simulink model "chou1"  (Simulink 2.09)
settings: Solver=ode45  StartTime=0.0  StopTime=9999  MaxStep=0.001  RelTol=1e-5  AbsTol=1e-5
settings Model: SaveTime=off  SaveOutput=off  ConsistencyChecking=off  RTWTemplateMakefile=grt_vc.tmf

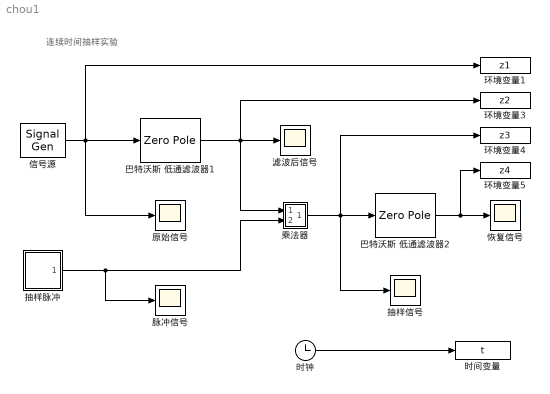
== system chou1 ==
  note: 连续时间抽样实验
  巴特沃斯 低通滤波器1 : ZeroPole  Zeros=z  Poles=p  Gain=k  mask(buttap){@1=60, @2=4}
      mask prompts: @1 "Cutoff frequency (rad/sec)"; @2 "Order"
      mask help:
      | Analog Butterworth low pass filter.
      |
      | (Requires Signal Processing Toolbox)
      mask init:
      | [z,p,k]=buttap(@2); z=@1*z; p=@1*p; k=real(prod(-p)); [num,den]=zp2tf(z,p,k); w=logspace(log10(@1/10),log10(10*@1),20); h=freqs(num,den,w);
      mask Help: Butterworth low pass filter using MATLAB's butter command.
      mask Display: plot(20*log10(w),20*log10(abs(h)))
  巴特沃斯 低通滤波器2 : ZeroPole  Zeros=z  Poles=p  Gain=k  mask(buttap){@1=60, @2=4}
      mask prompts: @1 "Cutoff frequency (rad/sec)"; @2 "Order"
      mask help:
      | Analog Butterworth low pass filter.
      |
      | (Requires Signal Processing Toolbox)
      mask init:
      | [z,p,k]=buttap(@2); z=@1*z; p=@1*p; k=real(prod(-p)); [num,den]=zp2tf(z,p,k); w=logspace(log10(@1/10),log10(10*@1),20); h=freqs(num,den,w);
      mask Help: Butterworth low pass filter using MATLAB's butter command.
      mask Display: plot(20*log10(w),20*log10(abs(h)))
  乘法器 : Subsystem
      mask Type: Dot Product
      mask Description:
      | Inner (dot) product.
      | y=sum(u1.*u2)
      mask Help: Computes the inner (dot) product of the inputs: sum(u1.*u2).  The inputs are vectors of the same length. Output is a scalar.
      mask Display: disp('X')
  抽样脉冲 : Subsystem  mask(Pulse Generator){@1=pi/100, @2=0.001, @3=1, @4=0.5}
      mask prompts: @1 "Pulse period (secs):"; @2 "Pulse width:"; @3 "Pulse height:"; @4 "Pulse start time:"
      mask help: Pulse Generator.
      mask init:
      | Ts=@1; du=@2; ht=@3; stt=@4; ini=ones(length(ht),1); st1=rem(stt,Ts); st2=rem(stt+du,Ts);if(Ts<=1.2*du),ini=zeros(length(ht),1);end;
      mask Help: Pulse generator which ensures pulse\ntransitions are hit. Provides a vector of pulses when the height is entered as a vector.\nUnmask to see how it works.
      mask Display: plot(0,0,100,100,[90,75,75,60,60,35,35,20,20,10],[20,20,80,80,20,20,80,80,20,20])
  抽样信号 : Scope
      settings: TickLabels=on  TimeRange=5  YMin=-2.6048  YMax=2.6048  SaveToWorkspace=off  SaveName=ScopeData
  环境变量1 : ToWorkspace  VariableName=z1  SampleTime=0
      settings: Buffer=1024*2
  环境变量3 : ToWorkspace  VariableName=z2  SampleTime=0
      settings: Buffer=1024*2
  环境变量4 : ToWorkspace  VariableName=z3  SampleTime=0
      settings: Buffer=1024*2
  环境变量5 : ToWorkspace  VariableName=z4  SampleTime=0
      settings: Buffer=1024*2
  恢复信号 : Scope
      settings: TickLabels=on  TimeRange=5  YMin=-0.108928  YMax=0.108928  SaveToWorkspace=off  SaveName=ScopeData
  滤波后信号 : Scope
      settings: TickLabels=on  TimeRange=5  YMin=-2.58112  YMax=2.58112  SaveToWorkspace=off  SaveName=ScopeData
  脉冲信号 : Scope
      settings: TickLabels=on  TimeRange=1  YMin=-1.55104  YMax=1.55104  SaveToWorkspace=off  SaveName=ScopeData
  时间变量 : ToWorkspace  VariableName=t  SampleTime=0
      settings: Buffer=2048
  时钟 : Clock
  信号源 : SignalGenerator  WaveForm=sine  Amplitude=2.000000  Frequency=3.140000  Units=rad/sec
  原始信号 : Scope
      settings: TickLabels=on  TimeRange=5  YMin=-4  YMax=4  SaveToWorkspace=off  SaveName=ScopeData
  wires:
  时钟/1 -> 时间变量/1
  巴特沃斯 低通滤波器2/1 -> 环境变量5/1, 恢复信号/1
  抽样脉冲/1(out_1) -> 脉冲信号/1, 乘法器/2(in_2)
  乘法器/1(out_1) -> 环境变量4/1, 抽样信号/1, 巴特沃斯 低通滤波器2/1
  巴特沃斯 低通滤波器1/1 -> 环境变量3/1, 滤波后信号/1, 乘法器/1(in_1)
  信号源/1 -> 环境变量1/1, 原始信号/1, 巴特沃斯 低通滤波器1/1

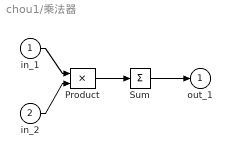
== system chou1/乘法器 ==
  in_1 : Inport  Port=1  PortWidth=-1  SampleTime=-1
  in_2 : Inport  Port=2  PortWidth=-1  SampleTime=-1
  Product : Product  Inputs=2
  Sum : Sum  Inputs=+
  out_1 : Outport  Port=1  InitialOutput=0
  wires:
  Sum/1 -> out_1/1
  Product/1 -> Sum/1
  in_1/1 -> Product/1
  in_2/1 -> Product/2

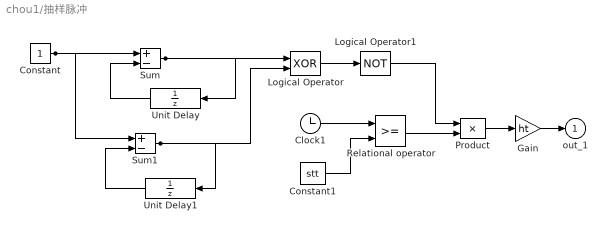
== system chou1/抽样脉冲 ==
  Clock1 : Clock
  Constant : Constant  Value=1
  Constant1 : Constant  Value=stt
  Gain : Gain  Gain=ht
  Logical Operator : Logic  Operator=XOR  Inputs=2
  Logical Operator1 : Logic  Operator=NOT  Inputs=1
  Product : Product  Inputs=2
  Relational operator : RelationalOperator  Operator=>=
  Sum : Sum  Inputs=+-
  Sum1 : Sum  Inputs=+-
  Unit Delay : UnitDelay  Orientation=left  X0=0  SampleTime=[Ts,st1]
  Unit Delay1 : UnitDelay  Orientation=left  X0=ini  SampleTime=[Ts,st2]
  out_1 : Outport  Port=1  InitialOutput=0
  wires:
  Sum1/1 -> Logical Operator/2, Unit Delay1/1
  Sum/1 -> Logical Operator/1, Unit Delay/1
  Constant/1 -> Sum1/1, Sum/1
  Unit Delay1/1 -> Sum1/2
  Unit Delay/1 -> Sum/2
  Clock1/1 -> Relational operator/1
  Relational operator/1 -> Product/2
  Product/1 -> Gain/1
  Gain/1 -> out_1/1
  Constant1/1 -> Relational operator/2
  Logical Operator/1 -> Logical Operator1/1
  Logical Operator1/1 -> Product/1
